simulink model "X_Ray_Control_System_stable_with_deadzone"  (R2025a)
settings: Solver=VariableStepAuto  StartTime=0.0  StopTime=10  RelTol=1e-3  EnableMultiTasking=on
model workspace (MAT data in the model file):
  Xtubecol = Simulink.Parameter
  Xtubecol.Value = [80 100 120]
  Xtubecol.Complexity = 'real'
  Xtubecol.Dimensions = [1 3]
  Xtubecol.DataType = 'auto'
  Xtuberow = Simulink.Parameter
  Xtuberow.Value = [3.327 3.3645 3.402 3.4395 3.477 3.5145 3.552 3.5895 3.627 3.6645 3.702 3.7395 3.777 3.8145 3.852 3.8895 3.927 3.9645 4.002 4.0395 4.077 4.1145 4.152 4.1895 4.227 4.2645 4.302 4.3395 4.377 4.4145 4.452 4.4895 4.527 4.5645 4.602 4.6395 4.677 4.7145 4.752 4.7895 4.827]
  Xtuberow.Complexity = 'real'
  Xtuberow.Dimensions = [1 41]
  Xtuberow.DataType = 'auto'
  Xtubet = Simulink.Parameter
  Xtubet.Value = [0  0  0; 1.24  1.52  1.79; 2.48  2.78  3.06; 3.71  4.03  4.34; 5  5.28  5.6; 6.19  6.54  6.89; 7.43  7.79  8.16; 8.66  9.05  9.44; 9.9  10.54  11.28; 12.94  12.8  13.57; 14.26  15.06  15.85; 16.48  17.32  18.14; 18.7  19.58  20.67; 21.44  22.86  24.26; 24.91  26.33  27.85; 28.38  29.91  31.9; 32.45  34.56  36.65; 37.06  39.25  41.72; 42.03  44.85  47.58; 47.67  50.73  54.07; 53.93  57.61  61.17; 60.72  65.1  69.15; 68.45  73.29  78.07; 76.9  80.23  87.76; 86.15  92.25  98.41; 96.25  103.13  110; 107.27  115.17  122.91; 119.34  128.07  136.92; 132.41  142.4  152.34; 146.8  157.87  168.86; 162.22  174.65  187; 179.09  192.82  206.76; 197.25  212.5  227.94; 216.76  233.82  250.65; 237.94  256.77  275.52; 260.65  281.38  302.22; 285.17  308.15  330.8; 311.48  336.54  361.74; 339.62  366.3  395; 369.6  400  431.34; 401.82  433.97  468.69]
  Xtubet.Complexity = 'real'
  Xtubet.Dimensions = [41 3]
  Xtubet.DataType = 'auto'
  tubefreq = Simulink.Parameter
  tubefreq.Value = 2
  tubefreq.Complexity = 'real'
  tubefreq.Dimensions = [1 1]
  tubefreq.DataType = 'auto'
  xtubecol = Simulink.Parameter
  xtubecol.Value = [80 100 120]
  xtubecol.Complexity = 'real'
  xtubecol.Dimensions = [1 3]
  xtubecol.DataType = 'auto'
  xtuberow = Simulink.Parameter
  xtuberow.Value = [3.327 3.3645 3.402 3.4395 3.477 3.5145 3.552 3.5895 3.627 3.6645 3.702 3.7395 3.777 3.8145 3.852 3.8895 3.927 3.9645 4.002 4.0395 4.077 4.1145 4.152 4.1895 4.227 4.2645 4.302 4.3395 4.377 4.4145 4.452 4.4895 4.527 4.5645 4.602 4.6395 4.677 4.7145 4.752 4.7895 4.827]
  xtuberow.Complexity = 'real'
  xtuberow.Dimensions = [1 41]
  xtuberow.DataType = 'auto'
  xtubet = Simulink.Parameter
  xtubet.Value = [0  0  0; 1.24  1.52  1.79; 2.48  2.78  3.06; 3.71  4.03  4.34; 5  5.28  5.6; 6.19  6.54  6.89; 7.43  7.79  8.16; 8.66  9.05  9.44; 9.9  10.54  11.28; 12.94  12.8  13.57; 14.26  15.06  15.85; 16.48  17.32  18.14; 18.7  19.58  20.67; 21.44  22.86  24.26; 24.91  26.33  27.85; 28.38  29.91  31.9; 32.45  34.56  36.65; 37.06  39.25  41.72; 42.03  44.85  47.58; 47.67  50.73  54.07; 53.93  57.61  61.17; 60.72  65.1  69.15; 68.45  73.29  78.07; 76.9  80.23  87.76; 86.15  92.25  98.41; 96.25  103.13  110; 107.27  115.17  122.91; 119.34  128.07  136.92; 132.41  142.4  152.34; 146.8  157.87  168.86; 162.22  174.65  187; 179.09  192.82  206.76; 197.25  212.5  227.94; 216.76  233.82  250.65; 237.94  256.77  275.52; 260.65  281.38  302.22; 285.17  308.15  330.8; 311.48  336.54  361.74; 339.62  366.3  395; 369.6  400  431.34; 401.82  433.97  468.69]
  xtubet.Complexity = 'real'
  xtubet.Dimensions = [41 3]
  xtubet.DataType = 'auto'
values from neighbouring files (symbols this model uses):
  fil_curr = [ ... (first row only)    [initialize_parameters.m]
  tube_curr_ref = [0:5:600]    [initialize_parameters.m]
  tube_kV_ref = [80:5:165]    [initialize_parameters.m]
  tubefreq = 2    [initialize_parameters.m]
undefined symbols (not defined in the file or in its folder): dspblkCoreblockFVToolHelper, gcbh
libraries: eeGeneralControl x1
settings Model: Creator=320180220  LastModifiedBy=320172975
settings SolverCC: PositivePriorityOrder=on
settings OptimizationCC: BlockReduction=off  ConditionallyExecuteInputs=off  DefaultParameterBehavior=Inlined  DefaultUnderspecifiedDataType=single  EnhancedBackFolding=on  PassReuseOutputArgsAs=Individual arguments  ZeroExternalMemoryAtStartup=off  ZeroInternalMemoryAtStartup=off  MaxStackSize=64  OptimizeBlockOrder=speed  DifferentSizesBufferReuse=on  OptimizationCustomize=off  EfficientTunableParamExpr=on
settings DebuggingCC: SingleTaskRateTransMsg=error  ParameterTunabilityLossMsg=error
settings HardwareCC: ProdBitPerPointer=32.0  ProdBitPerSizeT=32.0  ProdBitPerPtrDiffT=32.0  ProdLargestAtomicFloat=None  ProdIntDivRoundTo=Undefined  ProdEndianess=Unspecified  ProdWordSize=32.0  ProdHWDeviceType=ASIC/FPGA->ASIC/FPGA  TargetBitPerPointer=64.0  TargetBitPerSizeT=64.0  TargetBitPerPtrDiffT=64.0  TargetLongLongMode=on  TargetIntDivRoundTo=Zero  TargetEndianess=LittleEndian  TargetWordSize=64.0  TargetHWDeviceType=Custom Processor->MATLAB Host Computer  ProdEqTarget=off  HardwareBoardFeatureSet=SoCBlockset
settings ModelReferenceCC: ModelReferenceNumInstancesAllowed=Single
settings SFSimCC: MATLABDynamicMemAlloc=off
settings RTWCC: SystemTargetFile=ert.tlc  HardwareBoard=Altera Cyclone V SoC development kit  TLCOptions="-aInlineSetEventsForThisBaseRateFcn=TLC_FALSE -aSuppressMultiTaskScheduler=TLC_FALSE  -aRateBasedStepFcn=0"  TemplateMakefile=ert_default_tmf  GPUComputeCapability=3.5  Description=Embedded Coder
settings CodeAppCC: ForceParamTrailComments=on  IgnoreCustomStorageClasses=off  OperatorAnnotations=on  SimulinkDataObjDesc=on  SFDataObjDesc=on  InsertBlockDesc=on
settings ERTTargetCC: ExtModeTransport=0.0  ExtModeStaticAlloc=off  ExtModeMexFile=ext_comm  ExtModeIntrfLevel=Level1  SubcomponentCodeInterfacePackaging=Nonreusable function
settings ConfigComp: DVMaxProcessTime=300.0  DVMaxTestCaseSteps=10000.0  DVTestSuiteOptimization=Auto  DVAbsoluteTolerance=1.0e-5  DVDefectChecker=on  DVDetectOutOfBounds=on  DVMaxViolationSteps=20.0  DVModelReferenceHarness=on  DVHarnessSource=Signal Editor  DVActiveTab=0.0

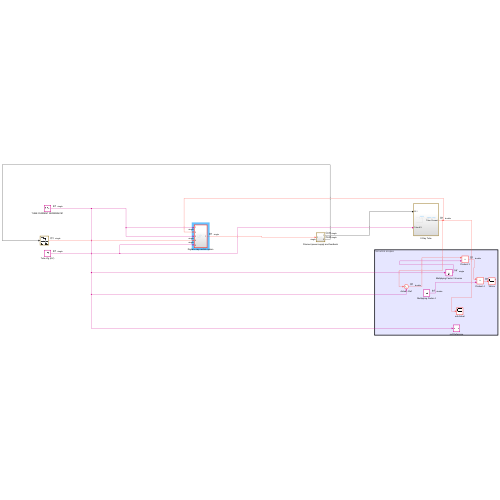
[thumbnail: Simulink's stored preview of the top-level diagram]
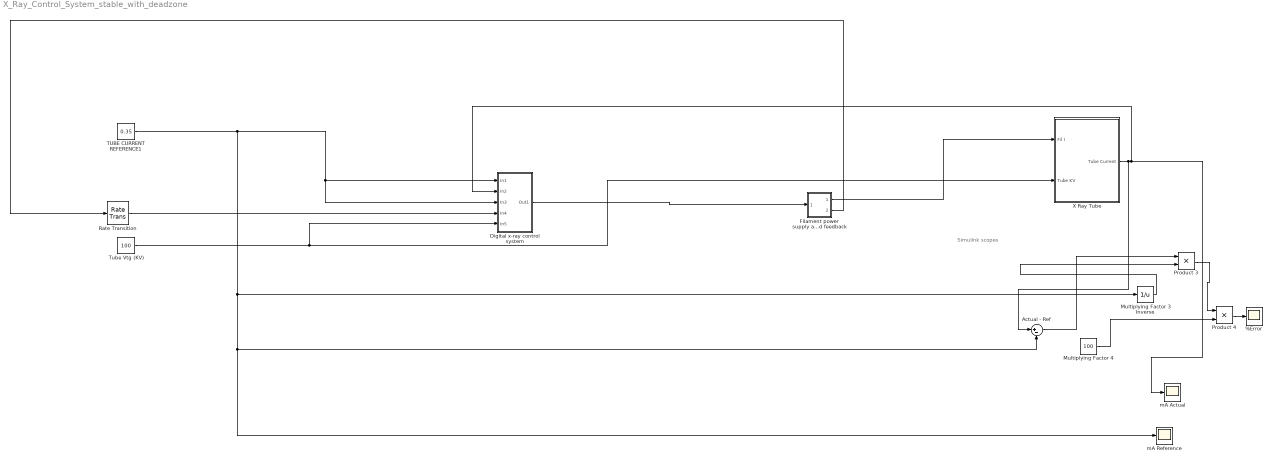
== system X_Ray_Control_System_stable_with_deadzone ==
  note: Simulink scopes
  %Error : Scope
      settings: ActiveDisplayYMinimum=-107.33103094252712  ActiveDisplayYMaximum=21.913640215940056  YLabel=Error %
  Actual - Ref : Sum  Inputs=|+-
  Digital x-ray control system : Subsystem  TreatAsAtomicUnit=on
  Filament power supply and feedback : Subsystem
  Multiplying Factor 3 Inverse : Math  Operator=reciprocal  SignedPower=on
  Multiplying Factor 4 : Constant  Value=100
  Product 3 : Product
  Product 4 : Product
  Rate Transition : RateTransition  OutPortSampleTime=0.01
  TUBE CURRENT REFERENCE1 : Constant  Value=0.35  OutDataTypeStr=single
  Tube Vtg (KV) : Constant  Value=100  OutDataTypeStr=single
  X Ray Tube : Subsystem
  mA Actual : Scope
      settings: ActiveDisplayYMinimum=-0.0479194458218592  ActiveDisplayYMaximum=0.513263329894381  YLabel=mA
  mA Reference : Scope
      settings: ActiveDisplayYMinimum=-0.72493810461173114  ActiveDisplayYMaximum=0.49734558772513943  YLabel=mA  DataLoggingVariableName=ScopeData2
  wires:
  Tube Vtg (KV)/1 -> X Ray Tube/2(Tube KV), Digital x-ray control system/5(In5)
  Digital x-ray control system/1(Out1) -> Filament power supply and feedback/1(In1)
  Filament power supply and feedback/1(Out1) -> X Ray Tube/1(Fil I)
  Filament power supply and feedback/2(Out2) -> Rate Transition/1
  X Ray Tube/1(Tube Current) -> mA Actual/1, Digital x-ray control system/2(In2), Actual - Ref/1
  Actual - Ref/1 -> Product 3/1
  TUBE CURRENT REFERENCE1/1 -> mA Reference/1, Actual - Ref/2, Multiplying Factor 3 Inverse/1, Digital x-ray control system/1(In1), Digital x-ray control system/3(In3)
  Product 3/1 -> Product 4/1
  Product 4/1 -> %Error/1
  Multiplying Factor 3 Inverse/1 -> Product 3/2
  Multiplying Factor 4/1 -> Product 4/2
  Rate Transition/1 -> Digital x-ray control system/4(In4)

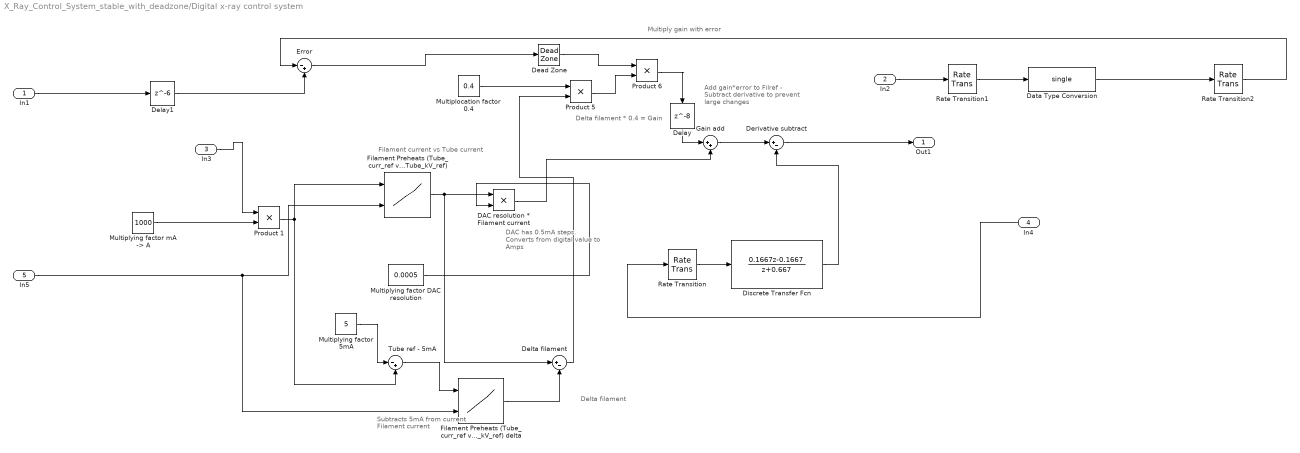
== system X_Ray_Control_System_stable_with_deadzone/Digital x-ray control system ==
  note: Add gain*error to Filref - Subtract derivative to prevent large changes
  note: Multiply gain with error
  note: Delta filament * 0.4 = Gain
  note: Delta filament
  note: Subtracts 5mA from current Filament current
  note: DAC has 0.5mA steps.
      | Converts from digital value to Amps
  note: Filament current vs Tube current
  In1 : Inport  OutDataTypeStr=single
  In2 : Inport  Port=2  SampleTime=0.01
  In3 : Inport  Port=3  OutDataTypeStr=single
  In4 : Inport  Port=4  OutDataTypeStr=single  SampleTime=0.01
  In5 : Inport  Port=5
  DAC resolution * Filament current : Product  OutDataTypeStr=single
  Data Type Conversion : DataTypeConversion  OutDataTypeStr=single  SaturateOnIntegerOverflow=off  RndMeth=Floor
  Dead Zone : DeadZone
  Delay : Delay  DelayLength=8
  Delay1 : Delay  DelayLength=6
  Delta filament : Sum  Inputs=|+-
  Derivative subtract : Sum  Inputs=|+-
  Discrete Transfer Fcn : DiscreteTransferFcn  LoadFcn=dspblkCoreblockFVToolHelper(gcbh,'load');  Numerator=[0.1667 -0.1667]  Denominator=[1 0.667]  OutDataTypeStr=Inherit: Same as input
      settings: CopyFcn=dspblkCoreblockFVToolHelper(gcbh,'copy');  DeleteFcn=dspblkCoreblockFVToolHelper(gcbh,'close');  ModelCloseFcn=dspblkCoreblockFVToolHelper(gcbh,'close');  PreSaveFcn=dspblkCoreblockFVToolHelper(gcbh,'presave');  PostSaveFcn=dspblkCoreblockFVToolHelper(gcbh,'postsave');  CloseFcn=dspblkCoreblockFVToolHelper(gcbh,'close');
  Error : Sum  Inputs=|-+
  Filament Preheats (Tube_curr_ref vs Tube_kV_ref) : Lookup_n-D  BreakpointsForDimension1=tube_curr_ref  BreakpointsForDimension2=tube_kV_ref  Table=fil_curr  InternalRulePriority=Speed  RndMeth=Simplest
      settings: InputPortMap=u0,u1
  Filament Preheats (Tube_curr_ref vs Tube_kV_ref) delta : Lookup_n-D  BreakpointsForDimension1=tube_curr_ref  BreakpointsForDimension2=tube_kV_ref  Table=fil_curr  InternalRulePriority=Speed  RndMeth=Simplest
      settings: InputPortMap=u0,u1
  Gain add : Sum  Inputs=|++
  Multiplocation factor 0.4 : Constant  Value=0.4  OutDataTypeStr=single
  Multiplying factor 5mA : Constant  Value=5  OutDataTypeStr=single
  Multiplying factor DAC resolution : Constant  Value=0.0005  OutDataTypeStr=single
  "Multiplying factor mA -> A" : Constant  Value=1000  OutDataTypeStr=single
  Product 1 : Product
  Product 5 : Product
  Product 6 : Product  OutDataTypeStr=single
  Rate Transition : RateTransition  OutPortSampleTime=0.01
  Rate Transition1 : RateTransition  OutPortSampleTime=0.01
  Rate Transition2 : RateTransition  OutPortSampleTime=0.01
  Tube ref - 5mA : Sum  Inputs=|-+
  Out1 : Outport
  wires:
  Delta filament/1 -> Product 5/2
  Multiplying factor DAC resolution/1 -> DAC resolution * Filament current/2
  Discrete Transfer Fcn/1 -> Derivative subtract/2
  DAC resolution * Filament current/1 -> Gain add/2
  Tube ref - 5mA/1 -> Filament Preheats (Tube_curr_ref vs Tube_kV_ref) delta/1
  Product 6/1 -> Delay/1
  Product 1/1 -> Filament Preheats (Tube_curr_ref vs Tube_kV_ref)/1, Tube ref - 5mA/2
  Product 5/1 -> Product 6/2
  Filament Preheats (Tube_curr_ref vs Tube_kV_ref) delta/1 -> Delta filament/2
  Multiplying factor 5mA/1 -> Tube ref - 5mA/1
  Dead Zone/1 -> Product 6/1
  Filament Preheats (Tube_curr_ref vs Tube_kV_ref)/1 -> Delta filament/1, DAC resolution * Filament current/1
  Multiplocation factor 0.4/1 -> Product 5/1
  Error/1 -> Dead Zone/1
  In4/1 -> Rate Transition/1
  "Multiplying factor mA -> A"/1 -> Product 1/2
  In5/1 -> Filament Preheats (Tube_curr_ref vs Tube_kV_ref) delta/2, Filament Preheats (Tube_curr_ref vs Tube_kV_ref)/2
  In2/1 -> Rate Transition1/1
  In3/1 -> Product 1/1
  In1/1 -> Delay1/1
  Derivative subtract/1 -> Out1/1
  Data Type Conversion/1 -> Rate Transition2/1
  Rate Transition/1 -> Discrete Transfer Fcn/1
  Rate Transition1/1 -> Data Type Conversion/1
  Rate Transition2/1 -> Error/1
  Gain add/1 -> Derivative subtract/1
  Delay/1 -> Gain add/1
  Delay1/1 -> Error/2

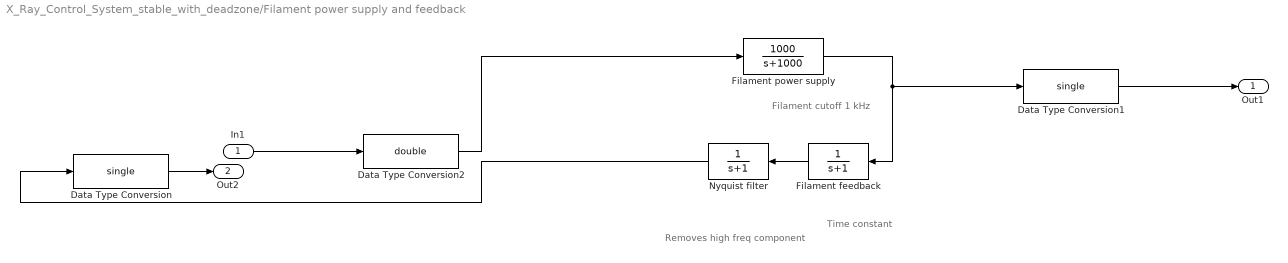
== system X_Ray_Control_System_stable_with_deadzone/Filament power supply and feedback ==
  note: Time constant
  note: Filament cutoff 1 kHz
  note: Removes high freq component
  In1 : Inport  OutDataTypeStr=single
  Data Type Conversion : DataTypeConversion  OutDataTypeStr=single  SaturateOnIntegerOverflow=off  RndMeth=Floor
  Data Type Conversion1 : DataTypeConversion  OutDataTypeStr=single  SaturateOnIntegerOverflow=off  RndMeth=Floor
  Data Type Conversion2 : DataTypeConversion  OutDataTypeStr=double  SaturateOnIntegerOverflow=off  RndMeth=Floor
  Filament feedback : TransferFcn  Denominator=[1 1]
  Filament power supply : TransferFcn  Numerator=[1000]  Denominator=[1 1000]
  Nyquist filter : TransferFcn  Denominator=[1 1]
  Out1 : Outport  OutDataTypeStr=single
  Out2 : Outport  Port=2  OutDataTypeStr=single
  wires:
  Filament power supply/1 -> Data Type Conversion1/1, Filament feedback/1
  In1/1 -> Data Type Conversion2/1
  Filament feedback/1 -> Nyquist filter/1
  Nyquist filter/1 -> Data Type Conversion/1
  Data Type Conversion/1 -> Out2/1
  Data Type Conversion1/1 -> Out1/1
  Data Type Conversion2/1 -> Filament power supply/1

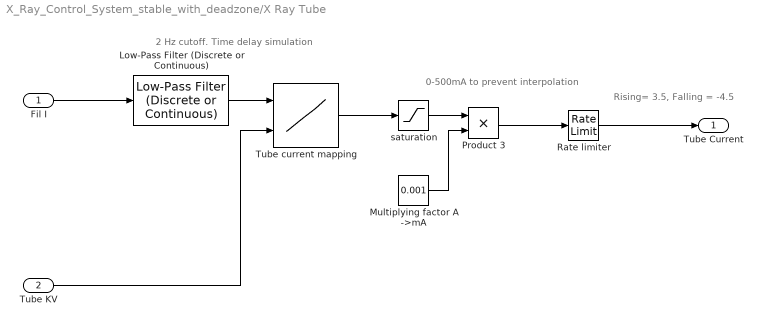
== system X_Ray_Control_System_stable_with_deadzone/X Ray Tube ==
  note: Rising= 3.5, Falling = -4.5
  note: 0-500mA to prevent interpolation
  note: 2 Hz cutoff. Time delay simulation
  Fil I : Inport
  Tube KV : Inport  Port=2
  Low-Pass Filter (Discrete or Continuous) : eeGeneralControl/Low-Pass Filter (Discrete or Continuous)  K=1  T=1/(2*pi*tubefreq)  B=inf  A=-inf  init_option=Specify as parameter  x0=0  Ts=-1
  Multiplying factor A ->mA : Constant  Value=0.001
  Product 3 : Product
  Rate limiter : RateLimiter  RisingSlewLimit=3.5  FallingSlewLimit=-4.5  SampleTimeMode=inherited
  Tube current mapping : Lookup_n-D  BreakpointsForDimension1=xtuberow  BreakpointsForDimension2=xtubecol  Table=xtubet  InternalRulePriority=Speed  RndMeth=Simplest
      settings: InputPortMap=u0,u1
  saturation : Saturate  UpperLimit=500  LowerLimit=0
  Tube Current : Outport
  wires:
  Low-Pass Filter (Discrete or Continuous)/1 -> Tube current mapping/1
  Tube current mapping/1 -> saturation/1
  Multiplying factor A ->mA/1 -> Product 3/2
  Rate limiter/1 -> Tube Current/1
  Product 3/1 -> Rate limiter/1
  saturation/1 -> Product 3/1
  Fil I/1 -> Low-Pass Filter (Discrete or Continuous)/1
  Tube KV/1 -> Tube current mapping/2
